simulink model "us_power_2022b"  (R2022b)
settings: Solver=VariableStepAuto  StartTime=0.0  StopTime=4  RelTol=1e-3
libraries: spsSeriesRLCBranchLib x6, spsCurrentMeasurementLib x3, spsVoltageMeasurementLib x3, slpidlib x2, spsIGBTDiodeLib x2, simulink x2, spsThreePhaseTransformerTwoWindingsLib x1, spsDCVoltageSourceLib x1, simulink_extras x1, eePwmGenerator x1, sps_lib x1, spsDiodeLib x1
settings Model: Creator=Administrator  LastModifiedBy=Administrator

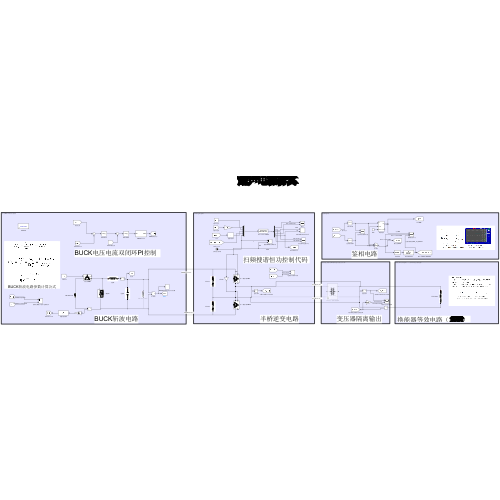
[thumbnail: Simulink's stored preview of the top-level diagram]
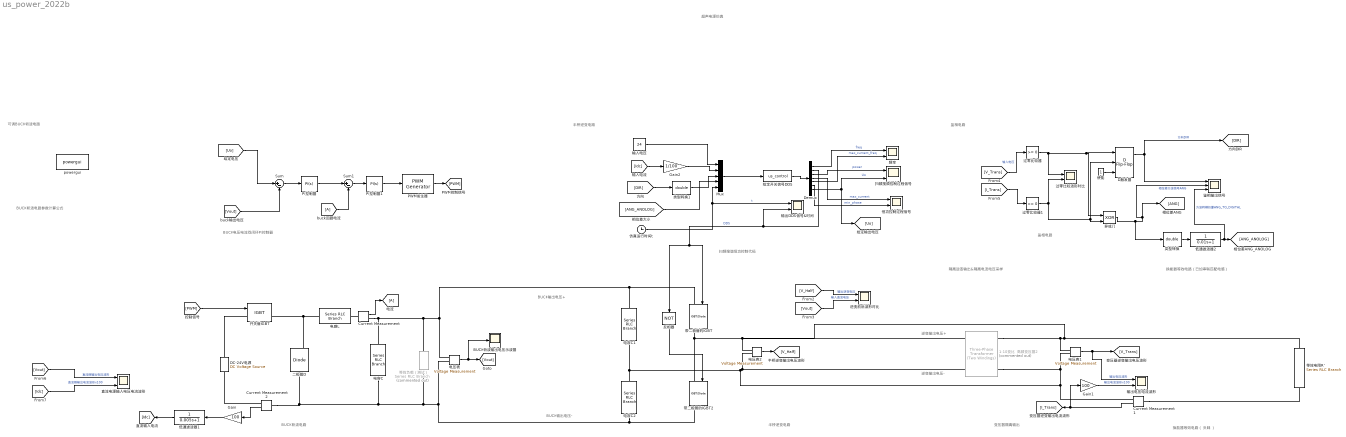
== system us_power_2022b ==
  note: 鉴相电路
  note: 换能器等效电路（已加串联匹配电感）
  note: 隔离逆变输出&隔离电流电压采样
  note: BUCK输出电压-
  note: BUCK输出电压+
  note: 半桥逆变电路
  note: 超声电源仿真
  note: BUCK斩波电路
  note: BUCK电压电流双闭环PI控制器
  note: BUCK斩波电路参数计算公式
  note: 可调BUCK斩波电路
  note: 半桥逆变电路
  note: 逆变输出电压+
  note: 逆变输出电压-
  note: 变压器隔离输出
  note: 换能器等效电路（ 负载 ）
  note: 扫频搜谐恒功控制代码
  note: 鉴相电路
  1:10变比  高频变压器2 : spsThreePhaseTransformerTwoWindingsLib/Three-Phase Transformer (Two Windings)  Commented=on  Winding1Connection=Yg  Winding2Connection=Yg  CoreType=Three single-phase transformers  SetSaturation=off  Hysteresis=off  DataFile='hysteresis'  SetInitialFlux=off  Measurements=None  UNITS=pu  NominalPower=[ 250e6 , 100]  Winding1=[ 100e3 , 0.002 , 0.02 ]  Winding2=[ 100e4 , 0.002 , 0.02]  Rm=500  Lm=500  L0=0.5  Saturation=[ 0,0 ; 0.0024,1.2 ; 1.0,1.52 ]  InitialFluxes=[ 0.8 , -0.8 , 0.7 ]  BreakLoop=off  DiscreteSolver=Trapezoidal iterative  DataType=off  TransfoNumber=1
  BUCK斩波输出电压示波器 : Scope
  Current Measurement : spsCurrentMeasurementLib/Current Measurement  PhasorSimulation=off  OutputType=Complex  PSBequivalent=0
  Current Measurement1 : spsCurrentMeasurementLib/Current Measurement  PhasorSimulation=off  OutputType=Complex  PSBequivalent=0
  Current Measurement2 : spsCurrentMeasurementLib/Current Measurement  PhasorSimulation=off  OutputType=Complex  PSBequivalent=0
  DC-24V电源 : spsDCVoltageSourceLib/DC Voltage Source  Amplitude=24  Measurements=None
  Demux : Demux  Outputs=7
  D触发器 : simulink_extras/Flip Flops/D Flip-Flop
  Gain : Gain  Gain=100
  Gain1 : Gain  Gain=100
  Gain2 : Gain  Gain=1/100
  Mux : Mux  Inputs=5
  PI控制器 : slpidlib/PID Controller  Controller=PI  Form=Parallel  TimeDomain=Continuous-time  UseExternalTs=off  SampleTime=-1  IntegratorMethod=Forward Euler  FilterMethod=Forward Euler  ControllerParametersSource=internal  P=1  I=10  UseKiTs=off  D=0  N=100  UseFilter=on  TunerSelectOption=Transfer Function Based (PID Tuner App)  InitialConditionSource=internal  InitialConditionForIntegrator=0  InitialConditionForFilter=0  DifferentiatorICPrevScaledInput=0  ExternalReset=none  TrackingMode=off  Kt=1  LimitOutput=off  SatLimitsSource=internal  UpperSaturationLimit=inf  LowerSaturationLimit=-inf  LinearizeAsGain=on  AntiWindupMode=none  Kb=1  LimitIntegrator=off  UpperIntegratorSaturationLimit=inf  LowerIntegratorSaturationLimit=-inf  POutMin=[]  POutMax=[]  IOutMin=[]  IOutMax=[]  DOutMin=[]  DOutMax=[]  NOutMin=[]  NOutMax=[]  SumOutMin=[]  SumOutMax=[]  SaturationOutMin=[]  SaturationOutMax=[]  PParamMin=[]  PParamMax=[]  IParamMin=[]  IParamMax=[]  DParamMin=[]  DParamMax=[]  NParamMin=[]  NParamMax=[]  KbParamMin=[]  KbParamMax=[]  KtParamMin=[]  KtParamMax=[]  KbOutMin=[]  KbOutMax=[]  KtOutMin=[]  KtOutMax=[]  IntegratorOutMin=[]  IntegratorOutMax=[]  FilterOutMin=[]  FilterOutMax=[]  SumI1OutMin=[]  SumI1OutMax=[]  SumI2OutMin=[]  SumI2OutMax=[]  SumI3OutMin=[]  SumI3OutMax=[]  SumI4OutMin=[]  SumI4OutMax=[]  SumDOutMin=[]  SumDOutMax=[]  DifferentiatorOutMin=[]  DifferentiatorOutMax=[]  FilterDiffOutCoefMin=[]  FilterDiffOutCoefMax=[]  ReciprocalOutMin=[]  ReciprocalOutMax=[]  SumDenOutMin=[]  SumDenOutMax=[]  SumNumOutMin=[]  SumNumOutMax=[]  DivideOutMin=[]  DivideOutMax=[]  UdiffTsProdOutMin=[]  UdiffTsProdOutMax=[]  NTsProdOutMin=[]  NTsProdOutMax=[]  UintegralTsProdOutMin=[]  UintegralTsProdOutMax=[]  UngainTsProdOutMin=[]  UngainTsProdOutMax=[]  ClampingZeroOutDataTypeStr=Inherit: Inherit via back propagation  ClampingZeroOutMin=[]  ClampingZeroOutMax=[]  FilterDenConstantOutDataTypeStr=Inherit: Inherit via back propagation  FilterDenConstantOutMin=[]  FilterDenConstantOutMax=[]  PCopyOutDataTypeStr=Inherit: Inherit via back propagation  PCopyOutMin=[]  PCopyOutMax=[]  NCopyOutDataTypeStr=Inherit: Inherit via back propagation  NCopyOutMin=[]  NCopyOutMax=[]  IntegratorContinuousStateAttributes=''  IntegratorStateMustResolveToSignalObject=off  IntegratorRTWStateStorageClass=Auto  FilterContinuousStateAttributes=''  FilterStateMustResolveToSignalObject=off  FilterRTWStateStorageClass=Auto  ParallelPVariant=InternalParameters  IdealPVariant=Disabled  IVariant=InternalParameters  DVariant=Disabled  IntegratorVariant=Continuous  SatVariant=Disabled  AWVariant=Passthrough  PCopyVariant=Disabled  TRVariant=Disabled  FdbkBlocksVariant=Forward  IdealPFdbkVariant=Disabled  SatFdbkVariant=Disabled  DerivativeFilterVariant=Disabled  NVariant=Disabled  NCopyVariant=Disabled_SignalSpec  FilterICVariant=Disabled  IntegratorICVariant=InternalICs  ExternalResetVariant=Disabled  TRSumVariant=Passthrough  SumFdbkVariant=Disabled  SumVariant=Sum_PI  TsampFilterVariant=InternalTs  TsampNgainVariant=Passthrough  TsampIntegralVariant=Passthrough  ExternalSaturationOutDataTypeStr=Inherit: Same as second input
  PI控制器1 : slpidlib/PID Controller  Controller=PI  Form=Parallel  TimeDomain=Continuous-time  UseExternalTs=off  SampleTime=-1  IntegratorMethod=Forward Euler  FilterMethod=Forward Euler  ControllerParametersSource=internal  P=1  I=1  UseKiTs=off  D=0  N=100  UseFilter=on  TunerSelectOption=Transfer Function Based (PID Tuner App)  InitialConditionSource=internal  InitialConditionForIntegrator=0  InitialConditionForFilter=0  DifferentiatorICPrevScaledInput=0  ExternalReset=none  TrackingMode=off  Kt=1  LimitOutput=off  SatLimitsSource=internal  UpperSaturationLimit=inf  LowerSaturationLimit=-inf  LinearizeAsGain=on  AntiWindupMode=none  Kb=1  LimitIntegrator=off  UpperIntegratorSaturationLimit=inf  LowerIntegratorSaturationLimit=-inf  POutMin=[]  POutMax=[]  IOutMin=[]  IOutMax=[]  DOutMin=[]  DOutMax=[]  NOutMin=[]  NOutMax=[]  SumOutMin=[]  SumOutMax=[]  SaturationOutMin=[]  SaturationOutMax=[]  PParamMin=[]  PParamMax=[]  IParamMin=[]  IParamMax=[]  DParamMin=[]  DParamMax=[]  NParamMin=[]  NParamMax=[]  KbParamMin=[]  KbParamMax=[]  KtParamMin=[]  KtParamMax=[]  KbOutMin=[]  KbOutMax=[]  KtOutMin=[]  KtOutMax=[]  IntegratorOutMin=[]  IntegratorOutMax=[]  FilterOutMin=[]  FilterOutMax=[]  SumI1OutMin=[]  SumI1OutMax=[]  SumI2OutMin=[]  SumI2OutMax=[]  SumI3OutMin=[]  SumI3OutMax=[]  SumI4OutMin=[]  SumI4OutMax=[]  SumDOutMin=[]  SumDOutMax=[]  DifferentiatorOutMin=[]  DifferentiatorOutMax=[]  FilterDiffOutCoefMin=[]  FilterDiffOutCoefMax=[]  ReciprocalOutMin=[]  ReciprocalOutMax=[]  SumDenOutMin=[]  SumDenOutMax=[]  SumNumOutMin=[]  SumNumOutMax=[]  DivideOutMin=[]  DivideOutMax=[]  UdiffTsProdOutMin=[]  UdiffTsProdOutMax=[]  NTsProdOutMin=[]  NTsProdOutMax=[]  UintegralTsProdOutMin=[]  UintegralTsProdOutMax=[]  UngainTsProdOutMin=[]  UngainTsProdOutMax=[]  ClampingZeroOutDataTypeStr=Inherit: Inherit via back propagation  ClampingZeroOutMin=[]  ClampingZeroOutMax=[]  FilterDenConstantOutDataTypeStr=Inherit: Inherit via back propagation  FilterDenConstantOutMin=[]  FilterDenConstantOutMax=[]  PCopyOutDataTypeStr=Inherit: Inherit via back propagation  PCopyOutMin=[]  PCopyOutMax=[]  NCopyOutDataTypeStr=Inherit: Inherit via back propagation  NCopyOutMin=[]  NCopyOutMax=[]  IntegratorContinuousStateAttributes=''  IntegratorStateMustResolveToSignalObject=off  IntegratorRTWStateStorageClass=Auto  FilterContinuousStateAttributes=''  FilterStateMustResolveToSignalObject=off  FilterRTWStateStorageClass=Auto  ParallelPVariant=InternalParameters  IdealPVariant=Disabled  IVariant=InternalParameters  DVariant=Disabled  IntegratorVariant=Continuous  SatVariant=Disabled  AWVariant=Passthrough  PCopyVariant=Disabled  TRVariant=Disabled  FdbkBlocksVariant=Forward  IdealPFdbkVariant=Disabled  SatFdbkVariant=Disabled  DerivativeFilterVariant=Disabled  NVariant=Disabled  NCopyVariant=Disabled_SignalSpec  FilterICVariant=Disabled  IntegratorICVariant=InternalICs  ExternalResetVariant=Disabled  TRSumVariant=Passthrough  SumFdbkVariant=Disabled  SumVariant=Sum_PI  TsampFilterVariant=InternalTs  TsampNgainVariant=Passthrough  TsampIntegralVariant=Passthrough  ExternalSaturationOutDataTypeStr=Inherit: Same as second input
  PWM发生器 : eePwmGenerator/PWM Generator  CarrCount=Up  Tper=0.001  Tdelay=0  Ts=5e-5
  Sum : Sum  Inputs=|+-
  Sum1 : Sum  Inputs=|+-
  buck回路电流 : From
  powergui : sps_lib/powergui  Priority=1  SimulationMode=Continuous  SampleTime=1e-5  frequency=60  Iterations=50  frequencyindice=0  Pbase=100e6  ErrMax=1e-4  UnitsV=kV  UnitsW=MW  buscounter=0  FunctionMessages=off  echomessages=off  EnableUseOfTLC=off  CurrentSourceSwitches=off  DisableSnubberDevices=off  DisableRonSwitches=off  DisableVfSwitches=off  DisplayEquations=off  AutomaticDiscreteSolvers=off  SolverType=Tustin/Backward Euler (TBE)  Interpol=off  ExternalGateDelay=off  methode=off  Ts=100  x0status=blocks  SPID=on  SwTol=0  HookPort=off  NonlinearTolerance=1e-4  nMaxIteration=100  ContinueOnMaxIteration=off  RestoreLinks=warning  ResistiveCurrentMeasurement=off  Frange=[0:2:500]  Ylog=off  Xlog=on  ShowGrid=off  save=off  variable=ZData  structure=0  ZoomFFT=off  StartTime=0.0  cycles=1  DisplayStyle=1  fundamental=60  FreqAxis=off  MaxFrequency=1000  frequencyindicesteady=1  RmsSteady=1  display=off
  二极管D : spsDiodeLib/Diode  Ron=0.001  Lon=0  Vf=0.8  IC=0  UseSnubber=0  Rs=500  Cs=250e-9  Measurements=on
  仿真运行时间t : Clock
  低通滤波器1 : TransferFcn  Denominator=[0.005 1]
  低通滤波器2 : TransferFcn  Denominator=[0.01 1]
  使能 : Constant
  反相器 : Logic  Operator=NOT  IconShape=distinctive  AllPortsSameDT=off  OutDataTypeStr=boolean
  带二极管的IGBT : spsIGBTDiodeLib/IGBT//Diode  Ron=1e-3  Rs=1e5  Cs=inf  Measurements=on
  带二极管的IGBT2 : spsIGBTDiodeLib/IGBT//Diode  Ron=1e-3  Rs=1e5  Cs=inf  Measurements=on
  开关管IGBT : spsIGBTLib/IGBT  Ron=0.001  Lon=0  Vf=1  Tf=1e-6  Tt=2e-6  IC=0  Rs=1e5  Cs=inf  Measurements=on
  异或门 : Logic  Operator=XOR  IconShape=distinctive  AllPortsSameDT=off  OutDataTypeStr=boolean
  恒功控制过程信号 : Scope  NumInputPorts=2
  扫频搜频控制过程信号 : Scope  NumInputPorts=2
  电压表 : spsVoltageMeasurementLib/Voltage Measurement  PhasorSimulation=off  OutputType=Complex  PSBequivalent=0
  电压表1 : spsVoltageMeasurementLib/Voltage Measurement  PhasorSimulation=off  OutputType=Complex  PSBequivalent=0
  电压表2 : spsVoltageMeasurementLib/Voltage Measurement  PhasorSimulation=off  OutputType=Complex  PSBequivalent=0
  电容C : spsSeriesRLCBranchLib/Series RLC Branch  LConnTagsString=__new0  RConnTagsString=__new0  BranchType=C  Resistance=1  Inductance=1e-3  SetiL0=off  InitialCurrent=0  Capacitance=470e-6  Setx0=on  InitialVoltage=0  Measurements=None
  电容C1 : spsSeriesRLCBranchLib/Series RLC Branch  LConnTagsString=__new0  RConnTagsString=__new0  BranchType=RC  Resistance=1  Inductance=1e-3  SetiL0=off  InitialCurrent=0  Capacitance=470e-6  Setx0=on  InitialVoltage=0  Measurements=None
  电容C2 : spsSeriesRLCBranchLib/Series RLC Branch  LConnTagsString=__new0  RConnTagsString=__new0  BranchType=RC  Resistance=1  Inductance=1e-3  SetiL0=off  InitialCurrent=0  Capacitance=470e-6  Setx0=on  InitialVoltage=0  Measurements=None
  电感L : spsSeriesRLCBranchLib/Series RLC Branch  LConnTagsString=__new0  RConnTagsString=__new0  BranchType=L  Resistance=1  Inductance=1e-3  SetiL0=off  InitialCurrent=0  Capacitance=1e-6  Setx0=off  InitialVoltage=0  Measurements=None
  电流 : Goto
  直流电源输入电压电流波形 : Scope  NumInputPorts=2
  "等效电阻R' " : spsSeriesRLCBranchLib/Series RLC Branch  LConnTagsString=__new0  RConnTagsString=__new0  BranchType=RLC  Resistance=10  Inductance=0.1  SetiL0=off  InitialCurrent=0  Capacitance=10e-6  Setx0=off  InitialVoltage=0  Measurements=None
  等效负载（测试） : spsSeriesRLCBranchLib/Series RLC Branch  Commented=on  LConnTagsString=__new0  RConnTagsString=__new0  BranchType=R  Resistance=100  Inductance=1e-3  SetiL0=off  InitialCurrent=0  Capacitance=1e-3  Setx0=on  InitialVoltage=0  Measurements=None
  类型转换 : DataTypeConversion  OutDataTypeStr=double  SaturateOnIntegerOverflow=off  RndMeth=Floor
  类型转换1 : DataTypeConversion  OutDataTypeStr=double  SaturateOnIntegerOverflow=off  RndMeth=Floor
  给定开关信号DDS : MATLABFcn  MATLABFcn=us_control  OutputDimensions=[1 7]  Output1D=off
  输入电压 : Constant  Value=24
  输出DDS信号&时间 : Scope  NumInputPorts=2
  输出电压电流波形 : Scope  NumInputPorts=2
  过零比较器 : simulink/Logic and Bit Operations/Compare To Zero  relop=>=  OutDataTypeStr=boolean
  过零比较器1 : simulink/Logic and Bit Operations/Compare To Zero  relop=>=  OutDataTypeStr=boolean
  过零比较波形对比 : Scope  NumInputPorts=2
  逆变前后波形对比 : Scope  NumInputPorts=2
  鉴相输出信号 : Scope  NumInputPorts=3
  频率 : Scope  NumInputPorts=2
  wires:
  [Uo] -> Sum/1
  [PWM] -> 开关管IGBT/1
  Sum1/1 -> PI控制器1/1
  buck回路电流/1 -> Sum1/2
  Current Measurement/1 -> 电流/1
  [Vout] -> Sum/2
  PI控制器/1 -> Sum1/1
  PWM发生器/1 -> [PWM]
  PI控制器1/1 -> PWM发生器/1
  Sum/1 -> PI控制器/1
  电压表/1 -> [Vout], BUCK斩波输出电压示波器/1
  反相器/1 -> 带二极管的IGBT2/1
  电压表2/1 -> [V_Half]
  电压表1/1 -> 输出电压电流波形/1, [V_Trans]  "输出电压波形"
  Current Measurement1/1 -> Gain1/1, [I_Trans]
  [Vout] -> 逆变前后波形对比/2  "输入直流电压"
  [V_Half] -> 逆变前后波形对比/1  "输出逆变电压"
  [I_Trans] -> 过零比较器1/1
  [V_Trans] -> 过零比较器/1  "输入电压"
  过零比较器1/1 -> D触发器/2, 异或门/2, 过零比较波形对比/2
  过零比较器/1 -> 异或门/1, D触发器/1, 过零比较波形对比/1
  异或门/1 -> 鉴相输出信号/2, [ANG], 类型转换/1  "相位差方波信号ANG"
  D触发器/1 -> [DIR], 鉴相输出信号/1  "方向DIR"
  使能/1 -> D触发器/3
  Gain1/1 -> 输出电压电流波形/2  "输出电流波形x100"
  Current Measurement2/1 -> Gain/1
  [Vout] -> 直流电源输入电压电流波形/1  "直流侧输出电压波形"
  输入电压/1 -> Mux/1
  [DIR] -> 类型转换1/1
  类型转换1/1 -> Mux/3
  [ANG_ANOLOG] -> Mux/4
  Mux/1 -> 给定开关信号DDS/1
  给定开关信号DDS/1 -> Demux/1
  [Idc] -> Gain2/1
  仿真运行时间t/1 -> 输出DDS信号&时间/1, Mux/5  "t"
  Demux/2 -> 输出DDS信号&时间/2, 反相器/1, 带二极管的IGBT/1  "DDS"
  类型转换/1 -> 低通滤波器2/1
  低通滤波器2/1 -> 鉴相输出信号/3, [ANG_ANOLOG]  "方波转模拟量ANG_TO_DIGITAL"
  Demux/1 -> 频率/1  "freq"
  Gain/1 -> 低通滤波器1/1
  [Idc] -> 直流电源输入电压电流波形/2  "直流侧输出电流波形x100"
  Demux/3 -> 扫频搜频控制过程信号/1  "power"
  Gain2/1 -> Mux/2
  Demux/4 -> 恒功控制过程信号/1  "max_current"
  Demux/6 -> 恒功控制过程信号/2  "min_phase"
  Demux/7 -> [Uo], 扫频搜频控制过程信号/2  "Uo"
  Demux/5 -> 频率/2  "max_current_freq"
  低通滤波器1/1 -> [Idc]
  connections:
  开关管IGBT/RConn1 -- 电感L/LConn1 -- 二极管D/RConn1
  电容C1/LConn1 -- 带二极管的IGBT/LConn1 -- 等效负载（测试）/LConn1 -- Current Measurement/RConn1 -- 电容C/LConn1 -- 电压表/LConn1
  电容C2/RConn1 -- 电压表/LConn2 -- 等效负载（测试）/RConn1 -- 电容C/RConn1 -- Current Measurement2/LConn1 -- 二极管D/LConn1 -- 带二极管的IGBT2/RConn1
  DC-24V电源/RConn1 -- 开关管IGBT/LConn1
  Current Measurement/LConn1 -- 电感L/RConn1
  Current Measurement1/LConn1 -- "等效电阻R' "/RConn1
  Current Measurement2/RConn1 -- DC-24V电源/LConn1
  电容C2/LConn1 -- 1:10变比  高频变压器2/RConn3 -- 电压表1/LConn2 -- Current Measurement1/RConn1 -- 1:10变比  高频变压器2/LConn3 -- 电压表2/LConn2 -- 电容C1/RConn1
  带二极管的IGBT2/LConn1 -- 1:10变比  高频变压器2/RConn1 -- 电压表1/LConn1 -- "等效电阻R' "/LConn1 -- 1:10变比  高频变压器2/LConn1 -- 电压表2/LConn1 -- 带二极管的IGBT/RConn1
